simulink model "Problem_3"  (R2020a)
settings: Solver=ode45  StartTime=0.0  StopTime=120  RelTol=1e-3
PreLoadFcn:
  | Kp=22;
  | Ki=4.5;
  | Kd=3.6;
  | m = 1000 ;
  | b = 50 ;
  | u = 500;
settings Model: Creator=Ganesh  LastModifiedBy=Ganesh

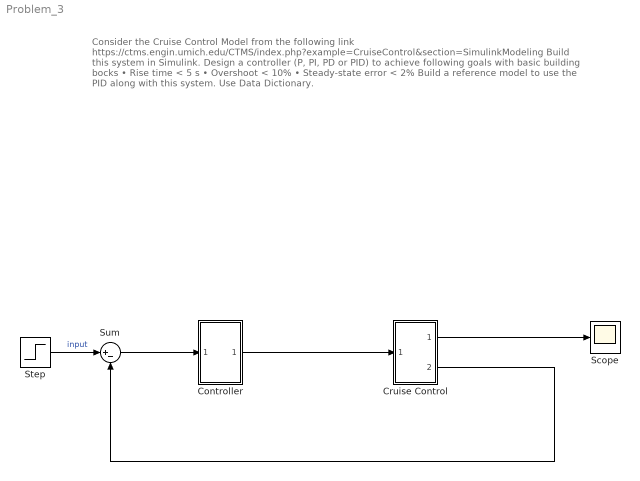
== system Problem_3 ==
  note: Consider the Cruise Control Model from the following link
      | https://ctms.engin.umich.edu/CTMS/index.php?example=CruiseControl&section=SimulinkModeling Build this system in Simulink.
      | Design a controller (P, PI, PD or PID) to achieve following goals with basic building bocks
      | • Rise time < 5 s
      | • Overshoot < 10%
      | • Steady-state error < 2%
      | Build a reference model to use the PID along with this system. Use Data Dictionary.
  Controller : Subsystem
  Cruise Control : Subsystem
  Scope : Scope
  Step : Step  Time=0  After=u  SampleTime=0
  Sum : Sum  Inputs=|+-
  wires:
  Step/1 -> Sum/1  "input"
  Sum/1 -> Controller/1(In1)
  Controller/1(Out1) -> Cruise Control/1(In1)
  Cruise Control/1(output) -> Scope/1
  Cruise Control/2(Out2) -> Sum/2

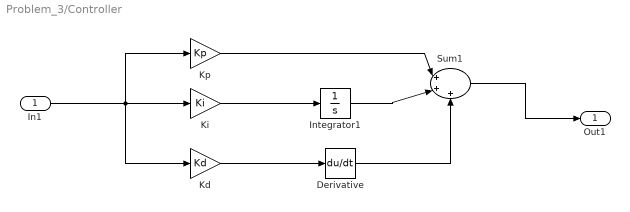
== system Problem_3/Controller ==
  In1 : Inport  OutDataTypeStr=double  PortDimensions=1  SampleTime=0
  Derivative : Derivative
  Integrator1 : Integrator
  Kd : Gain  Gain=Kd
  Ki : Gain  Gain=Ki
  Kp : Gain  Gain=Kp
  Sum1 : Sum  Inputs=|+++
  Out1 : Outport  OutDataTypeStr=double  PortDimensions=1  SampleTime=0
  wires:
  Kp/1 -> Sum1/1
  Integrator1/1 -> Sum1/2
  Kd/1 -> Derivative/1
  In1/1 -> Kp/1, Ki/1, Kd/1
  Derivative/1 -> Sum1/3
  Ki/1 -> Integrator1/1
  Sum1/1 -> Out1/1

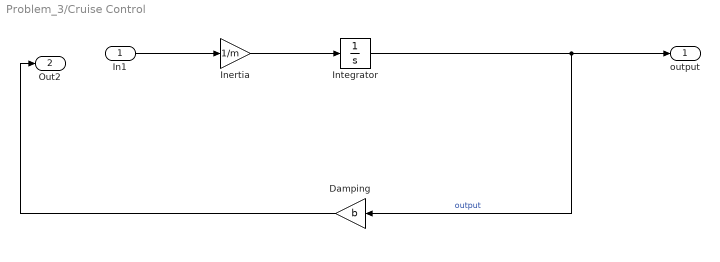
== system Problem_3/Cruise Control ==
  In1 : Inport
  Damping : Gain  Gain=b
  Inertia : Gain  Gain=1/m
  Integrator : Integrator
  output : Outport
  Out2 : Outport  Port=2
  wires:
  In1/1 -> Inertia/1
  Integrator/1 -> output/1, Damping/1  "output"
  Damping/1 -> Out2/1
  Inertia/1 -> Integrator/1
